simulink model "ejemplosim"  (R2017a)
settings: Solver=ode45  StartTime=0.0  StopTime=7  RelTol=1e-3  EnableMultiTasking=on
settings Model: Creator=Administrador  LastModifiedBy=Administrador
settings DataIOCC: LimitDataPoints=on  SaveFormat=Array
settings OptimizationCC: LifeSpan=inf
settings DebuggingCC: SFUnexpectedBacktrackingDiag=warning  SFNoUnconditionalDefaultTransitionDiag=warning  SFExecutionAtInitializationDiag=none
settings HardwareCC: ProdBitPerPointer=32  ProdBitPerSizeT=32  ProdBitPerPtrDiffT=32  ProdLargestAtomicFloat=None  ProdIntDivRoundTo=Undefined  ProdEndianess=Unspecified  ProdWordSize=32  ProdHWDeviceType=32-bit Generic
settings ModelReferenceCC: PropagateSignalLabelsOutOfModel=off
settings GRTTargetCC: TargetLangStandard=C89/C90 (ANSI)  GeneratePreprocessorConditionals=Disable all
settings ConfigComp: CovMetricSettings=dw  CovHtmlReporting=on  CovSaveCumulativeToWorkspaceVar=on  CovSaveSingleToWorkspaceVar=on  CovExternalEMLEnable=off

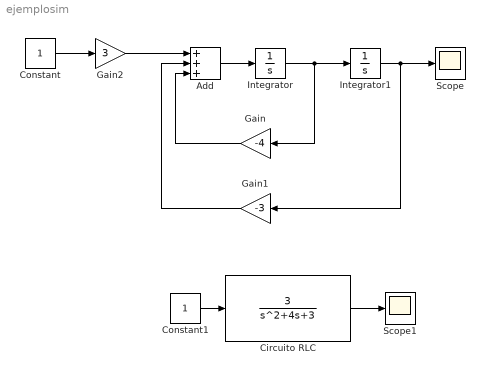
== system ejemplosim ==
  Add : Sum  Inputs=+++
  Circuito RLC : TransferFcn  Numerator=[3]  Denominator=[1 4 3]
  Constant : Constant
  Constant1 : Constant
  Gain : Gain  Gain=-4
  Gain1 : Gain  Gain=-3
  Gain2 : Gain  Gain=3
  Integrator : Integrator
  Integrator1 : Integrator
  Scope : Scope
  Scope1 : Scope
  wires:
  Integrator/1 -> Gain/1, Integrator1/1
  Add/1 -> Integrator/1
  Gain/1 -> Add/3
  Gain1/1 -> Add/2
  Constant/1 -> Gain2/1
  Gain2/1 -> Add/1
  Integrator1/1 -> Scope/1, Gain1/1
  Constant1/1 -> Circuito RLC/1
  Circuito RLC/1 -> Scope1/1
